simulink model "SensorPlanta"  (Simulink 8.9)
settings: Solver=ode3  StartTime=0.0  StopTime=inf  RelTol=1e-3  EnableMultiTasking=on
undefined symbols (not defined in the file or in its folder): daq
libraries: daqlib x6
settings Model: Creator=nuevo  LastModifiedBy=Control Digital
settings OptimizationCC: ExpressionDepthLimit=2147483647
settings DebuggingCC: SolverPrmCheckMsg=warning

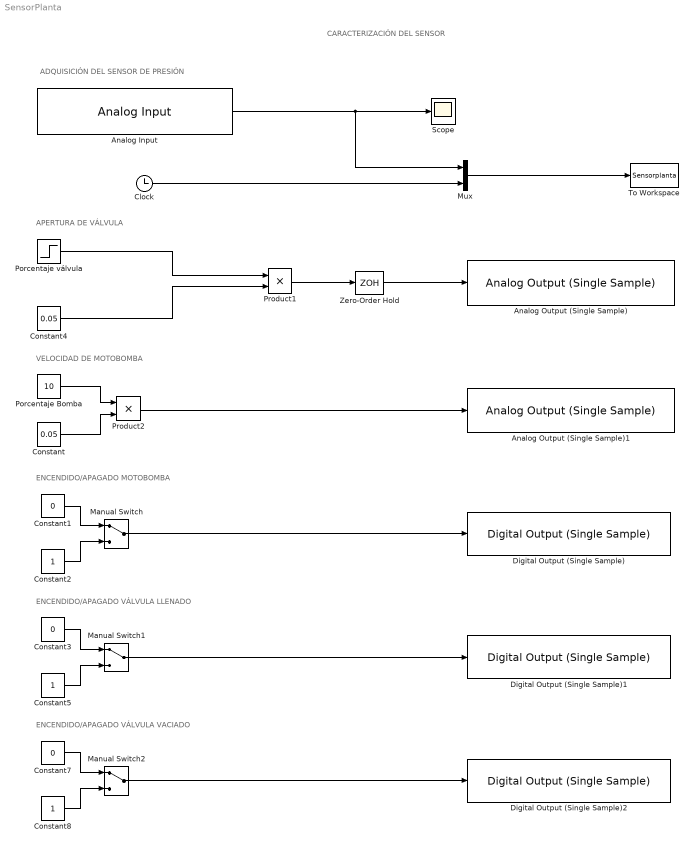
== system SensorPlanta ==
  note: CARACTERIZACIÓN DEL SENSOR
  note: VELOCIDAD DE MOTOBOMBA
  note: APERTURA DE VÁLVULA
  note: ENCENDIDO/APAGADO VÁLVULA VACIADO
  note: ENCENDIDO/APAGADO MOTOBOMBA
  note: ENCENDIDO/APAGADO VÁLVULA LLENADO
  note: ADQUISICIÓN DEL SENSOR DE PRESIÓN
  Analog Input : daqlib/Analog Input  DeviceMenu=ni Dev2 (USB-6009)  Device=ni Dev2 (USB-6009)  ObjConstructor=daq.createSession('ni')  NChannelsSelected=1  Channels=1$ai0$$Dev2$1$8$2$1$#0$ai1$$Dev2$1$8$2$1$#0$ai2$$Dev2$1$8$2$1$#0$ai3$$Dev2$1$8$2$1$#0$ai4$$Dev2$1$7$1$1$#0$ai5$$Dev2$1$7$1$1$#0$ai6$$Dev2$1$7$1$1$#0$ai7$$Dev2$1$7$1$1$#  NPorts=1 for all channels  SampleRate=5  ActualRate=5  ScansPerTrigger=50  OutputTimestamp=off  AcqMode=0  NumFrameBuffer=100  OutputTriggertime=off
      settings: SourceProductName=Data Acquisition Toolbox  SourceProductBaseCode=DA
  Analog Output (Single Sample) : daqlib/Analog Output (Single Sample)  DeviceMenu=ni Dev2 (USB-6009)  Device=ni Dev2 (USB-6009)  ObjConstructor=daq.createSession('ni')  NChannelsSelected=1  Channels=1$ao0$$Dev2$1$1$N/A$#0$ao1$$Dev2$1$1$N/A$#  NPorts=1 for all channels  BlockSampleTime=1
      settings: SourceProductName=Data Acquisition Toolbox  SourceProductBaseCode=DA
  Analog Output (Single Sample)1 : daqlib/Analog Output (Single Sample)  DeviceMenu=ni Dev2 (USB-6009)  Device=ni Dev2 (USB-6009)  ObjConstructor=daq.createSession('ni')  NChannelsSelected=1  Channels=0$ao0$$Dev2$1$1$N/A$#1$ao1$$Dev2$1$1$N/A$#  NPorts=1 for all channels  BlockSampleTime=1
      settings: SourceProductName=Data Acquisition Toolbox  SourceProductBaseCode=DA
  Clock : Clock
  Constant : Constant  Value=0.05
  Constant1 : Constant  Value=0  OutDataTypeStr=boolean
  Constant2 : Constant  OutDataTypeStr=boolean
  Constant3 : Constant  Value=0  OutDataTypeStr=boolean
  Constant4 : Constant  Value=0.05
  Constant5 : Constant  OutDataTypeStr=boolean
  Constant7 : Constant  Value=0  OutDataTypeStr=boolean
  Constant8 : Constant  OutDataTypeStr=boolean
  Digital Output (Single Sample) : daqlib/Digital Output (Single Sample)  DeviceMenu=ni Dev2 (USB-6009)  Device=ni Dev2 (USB-6009)  ObjConstructor=daq.createSession('ni')  BlockSampleTime=1  IsDigitalInput=off  NLinesSelected=1  Lines=1$port0/line0$$Dev2$#0$port0/line1$$Dev2$#0$port0/line2$$Dev2$#0$port0/line3$$Dev2$#0$port0/line4$$Dev2$#0$port0/line5$$Dev2$#0$port0/line6$$Dev2$#0$port0/line7$$Dev2$#0$port1/line0$$Dev2$#0$port1/line1$$Dev2$#0$port1/line2$$Dev2$#0$port1/line3$$Dev2$#  NPorts=1 for all lines
      settings: SourceProductName=Data Acquisition Toolbox  SourceProductBaseCode=DA
  Digital Output (Single Sample)1 : daqlib/Digital Output (Single Sample)  DeviceMenu=ni Dev2 (USB-6009)  Device=ni Dev2 (USB-6009)  ObjConstructor=daq.createSession('ni')  BlockSampleTime=1  IsDigitalInput=off  NLinesSelected=1  Lines=0$port0/line0$$Dev2$#1$port0/line1$$Dev2$#0$port0/line2$$Dev2$#0$port0/line3$$Dev2$#0$port0/line4$$Dev2$#0$port0/line5$$Dev2$#0$port0/line6$$Dev2$#0$port0/line7$$Dev2$#0$port1/line0$$Dev2$#0$port1/line1$$Dev2$#0$port1/line2$$Dev2$#0$port1/line3$$Dev2$#  NPorts=1 for all lines
      settings: SourceProductName=Data Acquisition Toolbox  SourceProductBaseCode=DA
  Digital Output (Single Sample)2 : daqlib/Digital Output (Single Sample)  DeviceMenu=ni Dev2 (USB-6009)  Device=ni Dev2 (USB-6009)  ObjConstructor=daq.createSession('ni')  BlockSampleTime=1  IsDigitalInput=off  NLinesSelected=1  Lines=0$port0/line0$$Dev2$#0$port0/line1$$Dev2$#1$port0/line2$$Dev2$#0$port0/line3$$Dev2$#0$port0/line4$$Dev2$#0$port0/line5$$Dev2$#0$port0/line6$$Dev2$#0$port0/line7$$Dev2$#0$port1/line0$$Dev2$#0$port1/line1$$Dev2$#0$port1/line2$$Dev2$#0$port1/line3$$Dev2$#  NPorts=1 for all lines
      settings: SourceProductName=Data Acquisition Toolbox  SourceProductBaseCode=DA
  Manual Switch : ManualSwitch
  Manual Switch1 : ManualSwitch
  Manual Switch2 : ManualSwitch
  Mux : Mux  Inputs=2
  Porcentaje Bomba : Constant  Value=10
  Porcentaje válvula : Step  After=50  SampleTime=0
  Product1 : Product  RndMeth=Zero
  Product2 : Product  RndMeth=Zero
  Scope : Scope
  To Workspace : ToWorkspace  VariableName=Sensorplanta  SampleTime=5
  Zero-Order Hold : ZeroOrderHold
  wires:
  Porcentaje válvula/1 -> Product1/1
  Constant7/1 -> Manual Switch2/1
  Porcentaje Bomba/1 -> Product2/1
  Product1/1 -> Zero-Order Hold/1
  Constant8/1 -> Manual Switch2/2
  Constant5/1 -> Manual Switch1/2
  Constant1/1 -> Manual Switch/1
  Constant3/1 -> Manual Switch1/1
  Constant2/1 -> Manual Switch/2
  Constant/1 -> Product2/2
  Constant4/1 -> Product1/2
  Product2/1 -> Analog Output (Single Sample)1/1
  Zero-Order Hold/1 -> Analog Output (Single Sample)/1
  Manual Switch/1 -> Digital Output (Single Sample)/1
  Manual Switch1/1 -> Digital Output (Single Sample)1/1
  Manual Switch2/1 -> Digital Output (Single Sample)2/1
  Clock/1 -> Mux/2
  Mux/1 -> To Workspace/1
  Analog Input/1 -> Scope/1, Mux/1
